simulink model "REL_TestModel"  (R2022a)
settings: Solver=FixedStepDiscrete  StartTime=0.0  StopTime=10.0  FixedStep=0.01  RelTol=1e-3
settings Model: DataDictionary=REL.sldd  Creator=DELL  LastModifiedBy=DELL
settings DataIOCC: SaveFormat=StructureWithTime
settings OptimizationCC: DefaultParameterBehavior=Inlined  EnhancedBackFolding=on  PassReuseOutputArgsAs=Individual arguments  ZeroExternalMemoryAtStartup=off  ZeroInternalMemoryAtStartup=off  OptimizeBlockOrder=speed  DifferentSizesBufferReuse=on  OptimizationCustomize=off  EfficientTunableParamExpr=on
settings DebuggingCC: ParameterTunabilityLossMsg=error
settings ModelReferenceCC: ModelReferenceNumInstancesAllowed=Single
settings SFSimCC: MATLABDynamicMemAlloc=off
settings RTWCC: Description=AUTOSAR  SystemTargetFile=autosar.tlc  GenCodeOnly=on  TemplateMakefile=ert_default_tmf
settings CodeAppCC: ForceParamTrailComments=on  IgnoreCustomStorageClasses=off  OperatorAnnotations=on  SimulinkDataObjDesc=on  SFDataObjDesc=on  InsertBlockDesc=on
settings STFCustomTargetCC: TargetLangStandard=C99 (ISO)  MultiwordLength=256  ParMdlRefBuildCompliant=on  CompOptLevelCompliant=on  IncludeMdlTerminateFcn=off  CombineOutputUpdateFcns=on  SuppressErrorStatus=on  ERTCustomFileBanners=on  SupportNonFinite=off  SupportComplex=off  SupportContinuousTime=off  SupportNonInlinedSFcns=off  RemoveResetFunc=on  MATLABClassNameForMDSCustomization=Simulink.SoftwareTarget.ERTCustomization  AutosarCompliant=on  GRTInterface=off  UseToolchainInfoCompliant=on  LookupTableObjectStructAxisOrder=2,1,3,4,...  LUTObjectStructOrderEvenSpacing=Size,Table,Breakpoints  SystemTargetFile=autosar.tlc
settings ERTTargetCC: TargetLangStandard=C99 (ISO)  ConcurrentExecutionCompliant=off  IncludeMdlTerminateFcn=off  SuppressErrorStatus=on  SupportNonFinite=off  SupportComplex=off  ModelStepFunctionPrototypeControlCompliant=off  CPPClassGenCompliant=off  AutosarCompliant=on  LookupTableObjectStructAxisOrder=2,1,3,4,...  LUTObjectStructOrderEvenSpacing=Size,Table,Breakpoints  InlinedParameterPlacement=NonHierarchical  ERTCustomFileTemplate=example_file_process.tlc

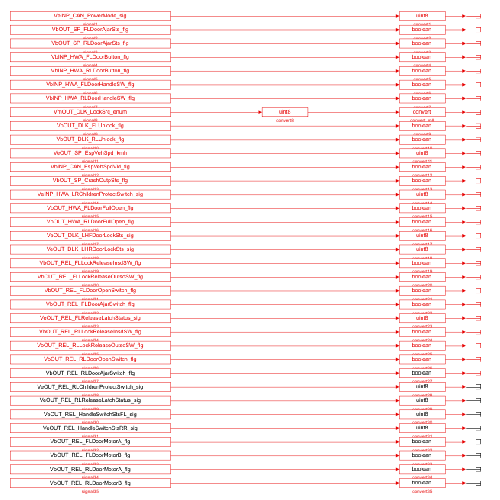
[thumbnail: Simulink's stored preview of the top-level diagram]
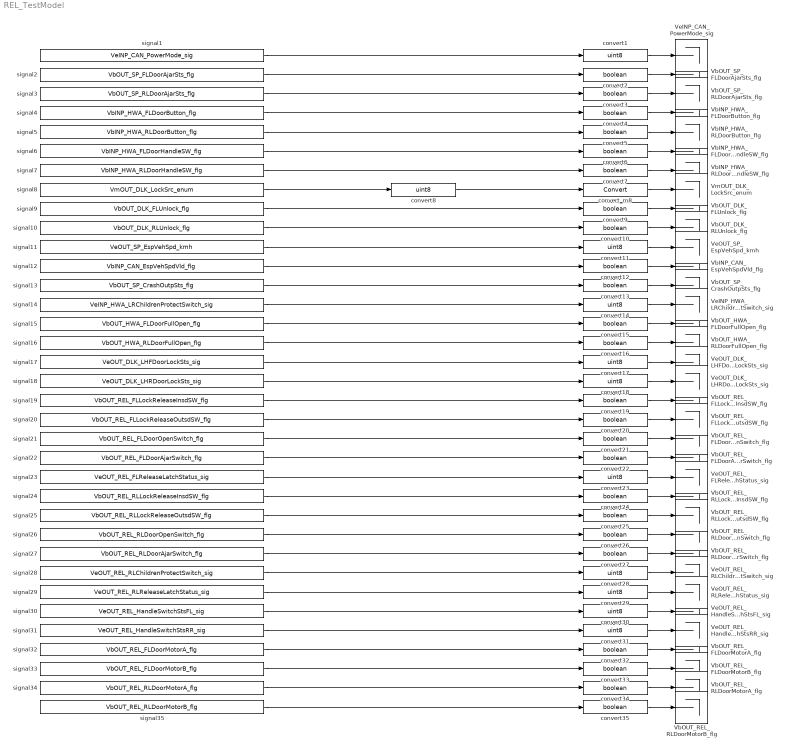
== system REL_TestModel ==
  VbINP_CAN_EspVehSpdVld_flg : Terminator
  VbINP_HWA_FLDoorButton_flg : Terminator
  VbINP_HWA_FLDoorHandleSW_flg : Terminator
  VbINP_HWA_RLDoorButton_flg : Terminator
  VbINP_HWA_RLDoorHandleSW_flg : Terminator
  VbOUT_DLK_FLUnlock_flg : Terminator
  VbOUT_DLK_RLUnlock_flg : Terminator
  VbOUT_HWA_FLDoorFullOpen_flg : Terminator
  VbOUT_HWA_RLDoorFullOpen_flg : Terminator
  VbOUT_REL_FLDoorAjarSwitch_flg : Terminator
  VbOUT_REL_FLDoorMotorA_flg : Terminator
  VbOUT_REL_FLDoorMotorB_flg : Terminator
  VbOUT_REL_FLDoorOpenSwitch_flg : Terminator
  VbOUT_REL_FLLockReleaseInsdSW_flg : Terminator
  VbOUT_REL_FLLockReleaseOutsdSW_flg : Terminator
  VbOUT_REL_RLDoorAjarSwitch_flg : Terminator
  VbOUT_REL_RLDoorMotorA_flg : Terminator
  VbOUT_REL_RLDoorMotorB_flg : Terminator
  VbOUT_REL_RLDoorOpenSwitch_flg : Terminator
  VbOUT_REL_RLLockReleaseInsdSW_flg : Terminator
  VbOUT_REL_RLLockReleaseOutsdSW_flg : Terminator
  VbOUT_SP_CrashOutpSts_flg : Terminator
  VbOUT_SP_FLDoorAjarSts_flg : Terminator
  VbOUT_SP_RLDoorAjarSts_flg : Terminator
  VeINP_CAN_PowerMode_sig : Terminator
  VeINP_HWA_LRChildrenProtectSwitch_sig : Terminator
  VeOUT_DLK_LHFDoorLockSts_sig : Terminator
  VeOUT_DLK_LHRDoorLockSts_sig : Terminator
  VeOUT_REL_FLReleaseLatchStatus_sig : Terminator
  VeOUT_REL_HandleSwitchStsFL_sig : Terminator
  VeOUT_REL_HandleSwitchStsRR_sig : Terminator
  VeOUT_REL_RLChildrenProtectSwitch_sig : Terminator
  VeOUT_REL_RLReleaseLatchStatus_sig : Terminator
  VeOUT_SP_EspVehSpd_kmh : Terminator
  VmOUT_DLK_LockSrc_enum : Terminator
  convert{1,8,11,14,17..18,23,28..31} (11 alike) : DataTypeConversion  OutDataTypeStr=uint8  SaturateOnIntegerOverflow=off  RndMeth=Floor
  convert{2..7,9..10,12..13,15..16,19..22,24..27,32..35} (24 alike) : DataTypeConversion  OutDataTypeStr=boolean  SaturateOnIntegerOverflow=off  RndMeth=Floor
  convert_m8 : DataTypeConversion  SaturateOnIntegerOverflow=off  RndMeth=Floor
  signal1 : FromWorkspace  VariableName=VeINP_CAN_PowerMode_sig  SampleTime=-1  Interpolate=off  OutputAfterFinalValue=Holding final value
  signal10 : FromWorkspace  VariableName=VbOUT_DLK_RLUnlock_flg  SampleTime=-1  Interpolate=off  OutputAfterFinalValue=Holding final value
  signal11 : FromWorkspace  VariableName=VeOUT_SP_EspVehSpd_kmh  SampleTime=-1  Interpolate=off  OutputAfterFinalValue=Holding final value
  signal12 : FromWorkspace  VariableName=VbINP_CAN_EspVehSpdVld_flg  SampleTime=-1  Interpolate=off  OutputAfterFinalValue=Holding final value
  signal13 : FromWorkspace  VariableName=VbOUT_SP_CrashOutpSts_flg  SampleTime=-1  Interpolate=off  OutputAfterFinalValue=Holding final value
  signal14 : FromWorkspace  VariableName=VeINP_HWA_LRChildrenProtectSwitch_sig  SampleTime=-1  Interpolate=off  OutputAfterFinalValue=Holding final value
  signal15 : FromWorkspace  VariableName=VbOUT_HWA_FLDoorFullOpen_flg  SampleTime=-1  Interpolate=off  OutputAfterFinalValue=Holding final value
  signal16 : FromWorkspace  VariableName=VbOUT_HWA_RLDoorFullOpen_flg  SampleTime=-1  Interpolate=off  OutputAfterFinalValue=Holding final value
  signal17 : FromWorkspace  VariableName=VeOUT_DLK_LHFDoorLockSts_sig  SampleTime=-1  Interpolate=off  OutputAfterFinalValue=Holding final value
  signal18 : FromWorkspace  VariableName=VeOUT_DLK_LHRDoorLockSts_sig  SampleTime=-1  Interpolate=off  OutputAfterFinalValue=Holding final value
  signal19 : FromWorkspace  VariableName=VbOUT_REL_FLLockReleaseInsdSW_flg  SampleTime=-1  Interpolate=off  OutputAfterFinalValue=Holding final value
  signal2 : FromWorkspace  VariableName=VbOUT_SP_FLDoorAjarSts_flg  SampleTime=-1  Interpolate=off  OutputAfterFinalValue=Holding final value
  signal20 : FromWorkspace  VariableName=VbOUT_REL_FLLockReleaseOutsdSW_flg  SampleTime=-1  Interpolate=off  OutputAfterFinalValue=Holding final value
  signal21 : FromWorkspace  VariableName=VbOUT_REL_FLDoorOpenSwitch_flg  SampleTime=-1  Interpolate=off  OutputAfterFinalValue=Holding final value
  signal22 : FromWorkspace  VariableName=VbOUT_REL_FLDoorAjarSwitch_flg  SampleTime=-1  Interpolate=off  OutputAfterFinalValue=Holding final value
  signal23 : FromWorkspace  VariableName=VeOUT_REL_FLReleaseLatchStatus_sig  SampleTime=-1  Interpolate=off  OutputAfterFinalValue=Holding final value
  signal24 : FromWorkspace  VariableName=VbOUT_REL_RLLockReleaseInsdSW_flg  SampleTime=-1  Interpolate=off  OutputAfterFinalValue=Holding final value
  signal25 : FromWorkspace  VariableName=VbOUT_REL_RLLockReleaseOutsdSW_flg  SampleTime=-1  Interpolate=off  OutputAfterFinalValue=Holding final value
  signal26 : FromWorkspace  VariableName=VbOUT_REL_RLDoorOpenSwitch_flg  SampleTime=-1  Interpolate=off  OutputAfterFinalValue=Holding final value
  signal27 : FromWorkspace  VariableName=VbOUT_REL_RLDoorAjarSwitch_flg  SampleTime=-1  Interpolate=off  OutputAfterFinalValue=Holding final value
  signal28 : FromWorkspace  VariableName=VeOUT_REL_RLChildrenProtectSwitch_sig  SampleTime=-1  Interpolate=off  OutputAfterFinalValue=Holding final value
  signal29 : FromWorkspace  VariableName=VeOUT_REL_RLReleaseLatchStatus_sig  SampleTime=-1  Interpolate=off  OutputAfterFinalValue=Holding final value
  signal3 : FromWorkspace  VariableName=VbOUT_SP_RLDoorAjarSts_flg  SampleTime=-1  Interpolate=off  OutputAfterFinalValue=Holding final value
  signal30 : FromWorkspace  VariableName=VeOUT_REL_HandleSwitchStsFL_sig  SampleTime=-1  Interpolate=off  OutputAfterFinalValue=Holding final value
  signal31 : FromWorkspace  VariableName=VeOUT_REL_HandleSwitchStsRR_sig  SampleTime=-1  Interpolate=off  OutputAfterFinalValue=Holding final value
  signal32 : FromWorkspace  VariableName=VbOUT_REL_FLDoorMotorA_flg  SampleTime=-1  Interpolate=off  OutputAfterFinalValue=Holding final value
  signal33 : FromWorkspace  VariableName=VbOUT_REL_FLDoorMotorB_flg  SampleTime=-1  Interpolate=off  OutputAfterFinalValue=Holding final value
  signal34 : FromWorkspace  VariableName=VbOUT_REL_RLDoorMotorA_flg  SampleTime=-1  Interpolate=off  OutputAfterFinalValue=Holding final value
  signal35 : FromWorkspace  VariableName=VbOUT_REL_RLDoorMotorB_flg  SampleTime=-1  Interpolate=off  OutputAfterFinalValue=Holding final value
  signal4 : FromWorkspace  VariableName=VbINP_HWA_FLDoorButton_flg  SampleTime=-1  Interpolate=off  OutputAfterFinalValue=Holding final value
  signal5 : FromWorkspace  VariableName=VbINP_HWA_RLDoorButton_flg  SampleTime=-1  Interpolate=off  OutputAfterFinalValue=Holding final value
  signal6 : FromWorkspace  VariableName=VbINP_HWA_FLDoorHandleSW_flg  SampleTime=-1  Interpolate=off  OutputAfterFinalValue=Holding final value
  signal7 : FromWorkspace  VariableName=VbINP_HWA_RLDoorHandleSW_flg  SampleTime=-1  Interpolate=off  OutputAfterFinalValue=Holding final value
  signal8 : FromWorkspace  VariableName=VmOUT_DLK_LockSrc_enum  SampleTime=-1  Interpolate=off  OutputAfterFinalValue=Holding final value
  signal9 : FromWorkspace  VariableName=VbOUT_DLK_FLUnlock_flg  SampleTime=-1  Interpolate=off  OutputAfterFinalValue=Holding final value
  wires:
  signal1/1 -> convert1/1
  signal2/1 -> convert2/1
  signal3/1 -> convert3/1
  signal4/1 -> convert4/1
  signal5/1 -> convert5/1
  signal6/1 -> convert6/1
  signal7/1 -> convert7/1
  signal8/1 -> convert8/1
  convert8/1 -> convert_m8/1
  signal9/1 -> convert9/1
  signal10/1 -> convert10/1
  signal11/1 -> convert11/1
  signal12/1 -> convert12/1
  signal13/1 -> convert13/1
  signal14/1 -> convert14/1
  signal15/1 -> convert15/1
  signal16/1 -> convert16/1
  signal17/1 -> convert17/1
  signal18/1 -> convert18/1
  signal19/1 -> convert19/1
  signal20/1 -> convert20/1
  signal21/1 -> convert21/1
  signal22/1 -> convert22/1
  signal23/1 -> convert23/1
  signal24/1 -> convert24/1
  signal25/1 -> convert25/1
  signal26/1 -> convert26/1
  signal27/1 -> convert27/1
  signal28/1 -> convert28/1
  signal29/1 -> convert29/1
  signal30/1 -> convert30/1
  signal31/1 -> convert31/1
  signal32/1 -> convert32/1
  signal33/1 -> convert33/1
  signal34/1 -> convert34/1
  signal35/1 -> convert35/1
  convert1/1 -> VeINP_CAN_PowerMode_sig/1
  convert10/1 -> VbOUT_DLK_RLUnlock_flg/1
  convert11/1 -> VeOUT_SP_EspVehSpd_kmh/1
  convert12/1 -> VbINP_CAN_EspVehSpdVld_flg/1
  convert13/1 -> VbOUT_SP_CrashOutpSts_flg/1
  convert14/1 -> VeINP_HWA_LRChildrenProtectSwitch_sig/1
  convert15/1 -> VbOUT_HWA_FLDoorFullOpen_flg/1
  convert16/1 -> VbOUT_HWA_RLDoorFullOpen_flg/1
  convert17/1 -> VeOUT_DLK_LHFDoorLockSts_sig/1
  convert18/1 -> VeOUT_DLK_LHRDoorLockSts_sig/1
  convert19/1 -> VbOUT_REL_FLLockReleaseInsdSW_flg/1
  convert2/1 -> VbOUT_SP_FLDoorAjarSts_flg/1
  convert20/1 -> VbOUT_REL_FLLockReleaseOutsdSW_flg/1
  convert21/1 -> VbOUT_REL_FLDoorOpenSwitch_flg/1
  convert22/1 -> VbOUT_REL_FLDoorAjarSwitch_flg/1
  convert23/1 -> VeOUT_REL_FLReleaseLatchStatus_sig/1
  convert24/1 -> VbOUT_REL_RLLockReleaseInsdSW_flg/1
  convert25/1 -> VbOUT_REL_RLLockReleaseOutsdSW_flg/1
  convert26/1 -> VbOUT_REL_RLDoorOpenSwitch_flg/1
  convert27/1 -> VbOUT_REL_RLDoorAjarSwitch_flg/1
  convert28/1 -> VeOUT_REL_RLChildrenProtectSwitch_sig/1
  convert29/1 -> VeOUT_REL_RLReleaseLatchStatus_sig/1
  convert3/1 -> VbOUT_SP_RLDoorAjarSts_flg/1
  convert30/1 -> VeOUT_REL_HandleSwitchStsFL_sig/1
  convert31/1 -> VeOUT_REL_HandleSwitchStsRR_sig/1
  convert32/1 -> VbOUT_REL_FLDoorMotorA_flg/1
  convert33/1 -> VbOUT_REL_FLDoorMotorB_flg/1
  convert34/1 -> VbOUT_REL_RLDoorMotorA_flg/1
  convert35/1 -> VbOUT_REL_RLDoorMotorB_flg/1
  convert4/1 -> VbINP_HWA_FLDoorButton_flg/1
  convert5/1 -> VbINP_HWA_RLDoorButton_flg/1
  convert6/1 -> VbINP_HWA_FLDoorHandleSW_flg/1
  convert7/1 -> VbINP_HWA_RLDoorHandleSW_flg/1
  convert9/1 -> VbOUT_DLK_FLUnlock_flg/1
  convert_m8/1 -> VmOUT_DLK_LockSrc_enum/1
